simulink model "models_BIBO"  (R2016a)
settings: Solver=VariableStepAuto  StartTime=0.0  StopTime=10  MaxStep=1e-2  RelTol=1e-3
libraries: simulink x1
settings Model: Creator=alexalcocer  LastModifiedBy=alepen

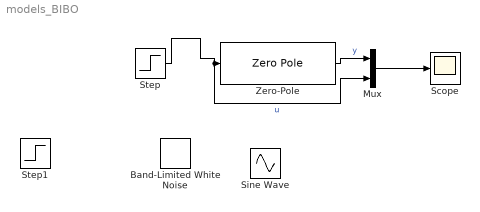
== system models_BIBO ==
  Band-Limited White Noise : simulink/Sources/Band-Limited White Noise  Cov=[0.1]  Ts=0.1  seed=[23341]
  Mux : Mux  Inputs=2
  Scope : Scope
  Sine Wave : Sin  SampleTime=0
  Step : Step  SampleTime=0
  Step1 : Step  SampleTime=0
  Zero-Pole : ZeroPole  Zeros=[-1 2]  Poles="[-2.3 1.2  -5.5]"
  wires:
  Mux/1 -> Scope/1
  Zero-Pole/1 -> Mux/1  "y"
  Step/1 -> Mux/2, Zero-Pole/1  "u"
